simulink model "Shema"  (R2024a)
settings: Solver=VariableStepAuto  StartTime=0.0  StopTime=10.0  RelTol=1e-3
undefined symbols (not defined in the file): K_lqr
settings Model: Creator=NB  LastModifiedBy=NB

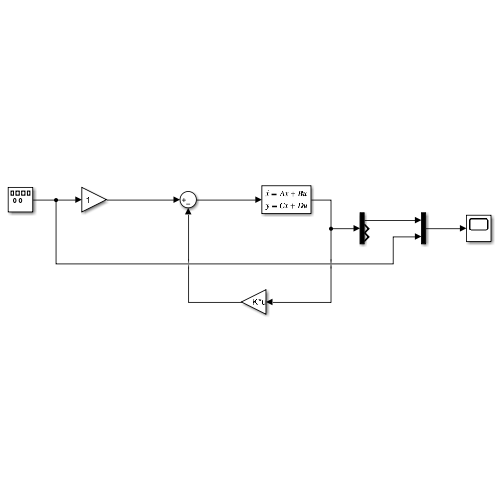
[thumbnail: Simulink's stored preview of the top-level diagram]
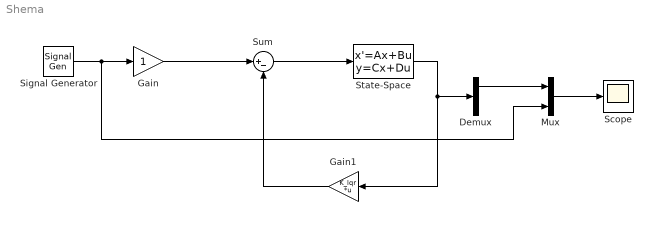
== system Shema ==
  Demux : Demux  Outputs=3
  Gain : Gain
  Gain1 : Gain  Gain=K_lqr  Multiplication=Matrix(K*u)
  Mux : Mux  Inputs=2
  Scope : Scope
  Signal Generator : SignalGenerator  WaveForm=square  Units=rad/sec
  State-Space : StateSpace  A=[0,1,0;0,-1.086513443191674,8.487176310246563e+03;0,-9.963636363636364e+03,-1.454545454545455e+06]  B=[0;0;3.636363636363637e+05]  C=[1,0,0; 0,1,0; 0,0,1]  D=[0; 0; 0]  InitialCondition=0
  Sum : Sum  Inputs=|+-
  wires:
  Signal Generator/1 -> Mux/2, Gain/1
  Gain/1 -> Sum/1
  Sum/1 -> State-Space/1
  State-Space/1 -> Demux/1, Gain1/1
  Gain1/1 -> Sum/2
  Demux/1 -> Mux/1
  Mux/1 -> Scope/1
